simulink model "RCS with Fans"  (R2025b)
settings: Solver=VariableStepAuto  StartTime=0.0  StopTime=30  FixedStep=0.1  RelTol=1e-3
libraries: slpidlib x1
settings Model: Creator=wangzerun  LastModifiedBy=wangzerun

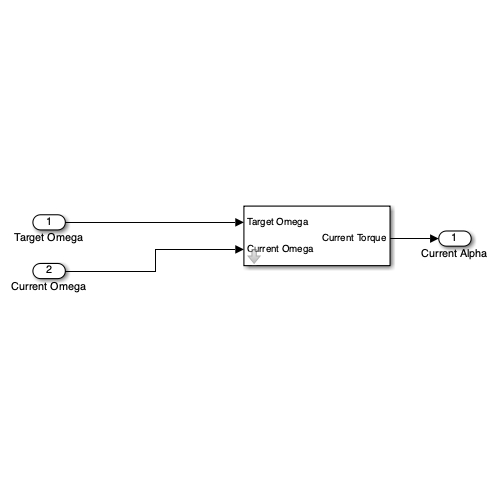
[thumbnail: Simulink's stored preview of the top-level diagram]
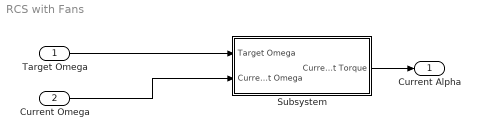
== system RCS with Fans ==
  Target Omega : Inport
  Current Omega : Inport  Port=2
  Subsystem : Subsystem  mask{max_thrust=3.53, idle_speed=0.15, radius=0.5}
      mask prompts: max_thrust "Max Thrust (N) (two motor total)"; idle_speed "Idle Speed (% of max speed in decimal)"; radius "Radius from fan installation point to center (m)"
  Current Alpha : Outport
  wires:
  Target Omega/1 -> Subsystem/1(Target Omega)
  Current Omega/1 -> Subsystem/2(Current Omega)
  Subsystem/1(Current Torque) -> Current Alpha/1

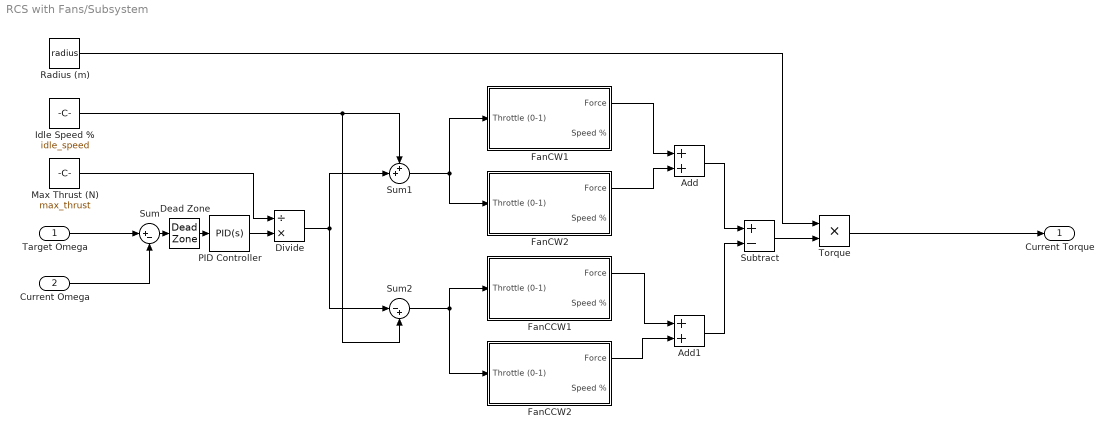
== system RCS with Fans/Subsystem ==
  Target Omega : Inport
  Current Omega : Inport  Port=2
  Add : Sum
  Add1 : Sum
  Dead Zone : DeadZone  LowerValue=-0.015  UpperValue=0.015
  Divide : Product  Inputs=/*
  FanCCW1 : Subsystem  mask{tau=0.1, F_max=3.53}
      mask prompts: tau "Time Constant (s)"; F_max "Max Thrust (N)"
  FanCCW2 : Subsystem  mask{tau=0.15, F_max=3.53}
      mask prompts: tau "Time Constant (s)"; F_max "Max Thrust (N)"
  FanCW1 : Subsystem  mask{tau=0.1, F_max=3.53}
      mask prompts: tau "Time Constant (s)"; F_max "Max Thrust (N)"
  FanCW2 : Subsystem  mask{tau=0.1, F_max=3.53}
      mask prompts: tau "Time Constant (s)"; F_max "Max Thrust (N)"
  Idle Speed % : Constant  Value=idle_speed
  Max Thrust (N) : Constant  Value=max_thrust
  PID Controller : slpidlib/PID Controller  Controller=PID  Form=Parallel  TimeDomain=Continuous-time  UseExternalTs=off  SampleTime=0.1  IntegratorMethod=Forward Euler  FilterMethod=Forward Euler  ControllerParametersSource=internal  P=2.5  I=1  UseKiTs=off  D=4  UseExternalDerivativeSource=off  N=2  UseFilter=on  TunerSelectOption=Transfer Function Based (PID Tuner App)  InitialConditionSource=internal  InitialConditionForIntegrator=0  InitialConditionForFilter=0  DifferentiatorICPrevScaledInput=0  ExternalReset=none  TrackingMode=off  Kt=1  LimitOutput=off  SatLimitsSource=internal  UpperSaturationLimit=inf  LowerSaturationLimit=-inf  LinearizeAsGain=on  AntiWindupMode=none  Kb=1  LimitIntegrator=off  UpperIntegratorSaturationLimit=inf  LowerIntegratorSaturationLimit=-inf  POutMin=[]  POutMax=[]  IOutMin=[]  IOutMax=[]  DOutMin=[]  DOutMax=[]  NOutMin=[]  NOutMax=[]  SumOutMin=[]  SumOutMax=[]  SaturationOutMin=[]  SaturationOutMax=[]  PParamMin=[]  PParamMax=[]  IParamMin=[]  IParamMax=[]  DParamMin=[]  DParamMax=[]  NParamMin=[]  NParamMax=[]  KbParamMin=[]  KbParamMax=[]  KtParamMin=[]  KtParamMax=[]  KbOutMin=[]  KbOutMax=[]  KtOutMin=[]  KtOutMax=[]  IntegratorOutMin=[]  IntegratorOutMax=[]  FilterOutMin=[]  FilterOutMax=[]  SumI1OutMin=[]  SumI1OutMax=[]  SumI2OutMin=[]  SumI2OutMax=[]  SumI3OutMin=[]  SumI3OutMax=[]  SumI4OutMin=[]  SumI4OutMax=[]  SumDOutMin=[]  SumDOutMax=[]  DifferentiatorOutMin=[]  DifferentiatorOutMax=[]  FilterDiffOutCoefMin=[]  FilterDiffOutCoefMax=[]  ReciprocalOutMin=[]  ReciprocalOutMax=[]  SumDenOutMin=[]  SumDenOutMax=[]  SumNumOutMin=[]  SumNumOutMax=[]  DivideOutMin=[]  DivideOutMax=[]  UdiffTsProdOutMin=[]  UdiffTsProdOutMax=[]  NTsProdOutMin=[]  NTsProdOutMax=[]  UintegralTsProdOutMin=[]  UintegralTsProdOutMax=[]  UngainTsProdOutMin=[]  UngainTsProdOutMax=[]  ClampingZeroOutDataTypeStr=Inherit: Inherit via back propagation  ClampingZeroOutMin=[]  ClampingZeroOutMax=[]  FilterDenConstantOutDataTypeStr=Inherit: Inherit via back propagation  FilterDenConstantOutMin=[]  FilterDenConstantOutMax=[]  PCopyOutDataTypeStr=Inherit: Inherit via back propagation  PCopyOutMin=[]  PCopyOutMax=[]  NCopyOutDataTypeStr=Inherit: Inherit via back propagation  NCopyOutMin=[]  NCopyOutMax=[]  IntegratorContinuousStateAttributes=''  IntegratorStateMustResolveToSignalObject=off  IntegratorRTWStateStorageClass=Auto  FilterContinuousStateAttributes=''  FilterStateMustResolveToSignalObject=off  FilterRTWStateStorageClass=Auto  ParallelPVariant=InternalParameters  IdealPVariant=Disabled  IVariant=InternalParameters  DVariant=InternalParameters  IntegratorVariant=Continuous  SatVariant=Disabled  AWVariant=Passthrough  PCopyVariant=Disabled  TRVariant=Disabled  FdbkBlocksVariant=Forward  IdealPFdbkVariant=Disabled  SatFdbkVariant=Disabled  DerivativeFilterVariant=ContFilter  NVariant=InternalParameters  NCopyVariant=Disabled  FilterICVariant=InternalICsFilter  IntegratorICVariant=InternalICs  ExternalResetVariant=Disabled  TRSumVariant=Passthrough  SumFdbkVariant=Disabled  SumVariant=Sum_PID  TsampFilterVariant=InternalTs  TsampNgainVariant=Passthrough  TsampIntegralVariant=Disabled_SignalSpec  ExternalSaturationOutDataTypeStr=Inherit: Same as second input  DerivativeSourceVariant=ErrorSignal  PreIntVariant=InternalPreInt
  Radius (m) : Constant  Value=radius
  Subtract : Sum  Inputs=+-
  Sum : Sum  Inputs=|+-
  Sum1 : Sum  Inputs=++|
  Sum2 : Sum  Inputs=|-+
  Torque : Product
  Current Torque : Outport
  wires:
  Torque/1 -> Current Torque/1
  Subtract/1 -> Torque/2
  Radius (m)/1 -> Torque/1
  Add1/1 -> Subtract/2
  FanCCW2/1(Force) -> Add1/2
  Add/1 -> Subtract/1
  Sum2/1 -> FanCCW2/1(Throttle (0-1)), FanCCW1/1(Throttle (0-1))
  FanCW1/1(Force) -> Add/1
  Idle Speed %/1 -> Sum2/2, Sum1/1
  Max Thrust (N)/1 -> Divide/1
  FanCCW1/1(Force) -> Add1/1
  PID Controller/1 -> Divide/2
  Sum/1 -> Dead Zone/1
  Divide/1 -> Sum2/1, Sum1/2
  Sum1/1 -> FanCW2/1(Throttle (0-1)), FanCW1/1(Throttle (0-1))
  Dead Zone/1 -> PID Controller/1
  Current Omega/1 -> Sum/2
  FanCW2/1(Force) -> Add/2
  Target Omega/1 -> Sum/1

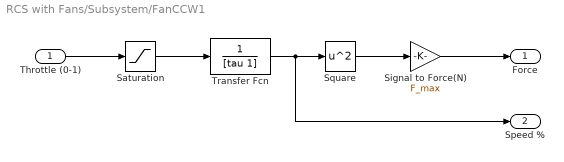
== system RCS with Fans/Subsystem/FanCCW1 ==
  Throttle (0-1) : Inport
  Saturation : Saturate  UpperLimit=1  LowerLimit=0.1
  Signal to Force(N) : Gain  Gain=F_max
  Square : Math  Operator=square
  Transfer Fcn : TransferFcn  Denominator=[tau 1]
  Force : Outport
  Speed % : Outport  Port=2
  wires:
  Saturation/1 -> Transfer Fcn/1
  Square/1 -> Signal to Force(N)/1
  Transfer Fcn/1 -> Speed %/1, Square/1
  Throttle (0-1)/1 -> Saturation/1
  Signal to Force(N)/1 -> Force/1

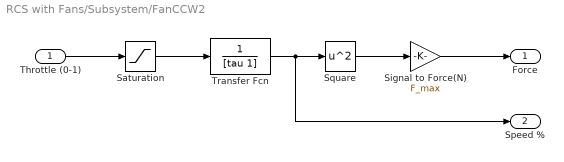
== system RCS with Fans/Subsystem/FanCCW2 ==
  Throttle (0-1) : Inport
  Saturation : Saturate  UpperLimit=1  LowerLimit=0.1
  Signal to Force(N) : Gain  Gain=F_max
  Square : Math  Operator=square
  Transfer Fcn : TransferFcn  Denominator=[tau 1]
  Force : Outport
  Speed % : Outport  Port=2
  wires:
  Saturation/1 -> Transfer Fcn/1
  Square/1 -> Signal to Force(N)/1
  Transfer Fcn/1 -> Speed %/1, Square/1
  Throttle (0-1)/1 -> Saturation/1
  Signal to Force(N)/1 -> Force/1

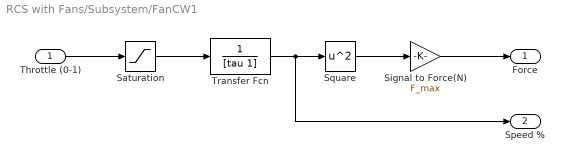
== system RCS with Fans/Subsystem/FanCW1 ==
  Throttle (0-1) : Inport
  Saturation : Saturate  UpperLimit=1  LowerLimit=0.1
  Signal to Force(N) : Gain  Gain=F_max
  Square : Math  Operator=square
  Transfer Fcn : TransferFcn  Denominator=[tau 1]
  Force : Outport
  Speed % : Outport  Port=2
  wires:
  Saturation/1 -> Transfer Fcn/1
  Square/1 -> Signal to Force(N)/1
  Transfer Fcn/1 -> Speed %/1, Square/1
  Throttle (0-1)/1 -> Saturation/1
  Signal to Force(N)/1 -> Force/1

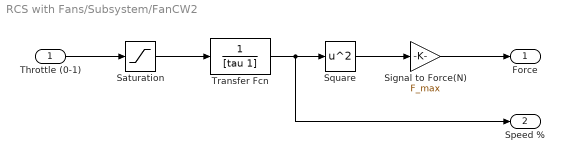
== system RCS with Fans/Subsystem/FanCW2 ==
  Throttle (0-1) : Inport
  Saturation : Saturate  UpperLimit=1  LowerLimit=0.1
  Signal to Force(N) : Gain  Gain=F_max
  Square : Math  Operator=square
  Transfer Fcn : TransferFcn  Denominator=[tau 1]
  Force : Outport
  Speed % : Outport  Port=2
  wires:
  Saturation/1 -> Transfer Fcn/1
  Square/1 -> Signal to Force(N)/1
  Transfer Fcn/1 -> Speed %/1, Square/1
  Throttle (0-1)/1 -> Saturation/1
  Signal to Force(N)/1 -> Force/1
